simulink model "Hall_sensor_120deg_bare"  (R2024b)
settings: Solver=FixedStepAuto  StartTime=0.0  StopTime=1  FixedStep=1e-6  RelTol=1e-3
values from neighbouring files (symbols this model uses):
  closed_loop = 0    [initialize_model.m]
  D_m = 1e-3    (= 0.001)    [initialize_model.m]
  hall_errors = [0 0 0]    [MTPA_sweep.m]    (also in initialize_model.m = (pi/180)*[-3,5,-4])
  J_t = 12e-4    (= 0.0012)    [initialize_model.m]
  L_ss = 0.45e-3    (= 0.00045)    [Arrow_86EMB3S98F_specs.m]    (also in M_2311P_specs.m = 0.0003657)
  lambda_m = 21.5e-3    (= 0.0215)    [Arrow_86EMB3S98F_specs.m]    (also in M_2311P_specs.m = 0.00985)
  P = 8    [Arrow_86EMB3S98F_specs.m]    (also in M_2311P_specs.m)
  r_s = 0.15    [Arrow_86EMB3S98F_specs.m]    (also in M_2311P_specs.m = 0.345)
  R_vs = 1e6    (= 1000000)    [initialize_model.m]
  T_m = torque_vals(i)    [MTPA_sweep.m]    (also in initialize_model.m = 1.53)
  tau_s = L_ss/r_s    (= 0.003)    [Arrow_86EMB3S98F_specs.m]    (also in M_2311P_specs.m = 0.00106)
  theta_v = pi/6    (= 0.523598775598)    [initialize_model.m]
  V_bus = 36    [initialize_model.m]
undefined symbols (not defined in the file or in its folder): DiscIntNeverNeededParam, dspblkCoreblockFVToolHelper, gcbh, HallError1, HallError2, HallError3, sysd, sysd_mech, WrappedHallError1
libraries: simulink x12, spsMosfetLib x6, spsSeriesRLCBranchLib x4, spsVoltageMeasurementLib x3, spsControlledCurrentSourceLib x3, embmathops x1, spsPWMGeneratorDCDCLib x1, spsDCVoltageSourceLib x1, sps_lib x1
settings Model: Creator=baolo  LastModifiedBy=baolo
settings DebuggingCC: IgnoredZcDiagnostic=none

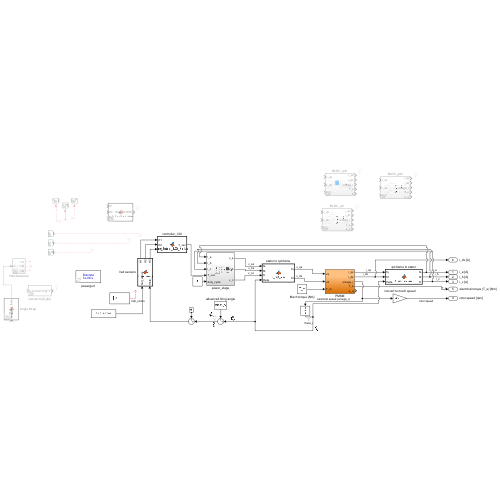
[thumbnail: Simulink's stored preview of the top-level diagram]
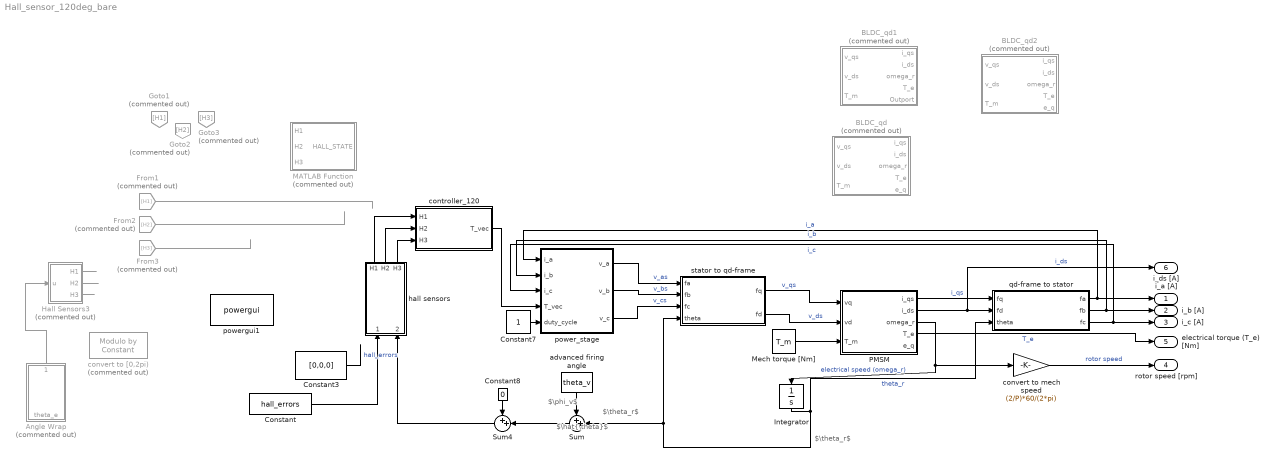
== system Hall_sensor_120deg_bare ==
  note: $\phi_v$
  note: $\theta_r$
  note: $\theta_r$
  note: $\hat{\theta}$
  Angle Wrap : MATLAB Function  Commented=on  TreatAsAtomicUnit=on
  BLDC_qd : Subsystem  Commented=on
  BLDC_qd1 : Subsystem  Commented=on
  BLDC_qd2 : Subsystem  Commented=on
  Constant : Constant  Value=hall_errors
  Constant3 : Constant  Value=[0,0,0]
  Constant7 : Constant
  Constant8 : Constant  Value=0
  From1 : From  Commented=on  GotoTag=H1
  From2 : From  Commented=on  GotoTag=H2
  From3 : From  Commented=on  GotoTag=H3
  Goto1 : Goto  Commented=on  GotoTag=H1
  Goto2 : Goto  Commented=on  GotoTag=H2
  Goto3 : Goto  Commented=on  GotoTag=H3
  Hall Sensors3 : Subsystem  Commented=on
  Integrator : Integrator
  MATLAB Function : MATLAB Function  Commented=on  TreatAsAtomicUnit=on
  Mech torque [Nm] : Constant  Value=T_m
  PMSM : Subsystem
  Sum : Sum  Inputs=++|
  Sum4 : Sum  Inputs=++|
  advanced firing angle : Constant  Value=theta_v
  controller_120 : MATLAB Function  TreatAsAtomicUnit=on
  convert to [0,2pi) : embmathops/Modulo by Constant  Commented=on  Denominator=2*pi  SimulateUsing=Code generation
      settings: LibrarySourceBlock=embeddedMathLib/Modulo by Constant
  convert to mech speed : Gain  Gain=(2/P)*60/(2*pi)
  hall sensors : MATLAB Function  TreatAsAtomicUnit=on
  power_stage : Subsystem
  powergui1 : sps_lib/powergui  Priority=1  SimulationMode=Discrete  SampleTime=1e-6  frequency=60  Iterations=50  frequencyindice=0  Pbase=100e6  ErrMax=1e-4  UnitsV=kV  UnitsW=MW  buscounter=0  FunctionMessages=off  echomessages=off  EnableUseOfTLC=off  CurrentSourceSwitches=off  DisableSnubberDevices=off  DisableRonSwitches=off  DisableVfSwitches=off  DisplayEquations=off  AutomaticDiscreteSolvers=off  SolverType=Tustin/Backward Euler (TBE)  Interpol=off  ExternalGateDelay=off  methode=off  Ts=100  x0status=blocks  SPID=on  SwTol=0  HookPort=off  NonlinearTolerance=1e-4  nMaxIteration=100  ContinueOnMaxIteration=off  RestoreLinks=warning  ResistiveCurrentMeasurement=off  Frange=[0:2:500]  Ylog=off  Xlog=on  ShowGrid=off  save=off  variable=ZData  structure=0  ZoomFFT=off  StartTime=0.0  cycles=1  DisplayStyle=1  fundamental=60  FreqAxis=off  MaxFrequency=1000  frequencyindicesteady=1  RmsSteady=1  display=off
  qd-frame to stator : MATLAB Function  TreatAsAtomicUnit=on
  stator to qd-frame : MATLAB Function  TreatAsAtomicUnit=on
  i_a [A] : Outport
  i_b [A] : Outport  Port=2
  i_c [A] : Outport  Port=3
  rotor speed [rpm] : Outport  Port=4
  electrical torque (T_e) [Nm] : Outport  Port=5
  i_ds [A] : Outport  Port=6
  wires:
  stator to qd-frame/1(fq) -> PMSM/1(vq)  "v_qs"
  stator to qd-frame/2(fd) -> PMSM/2(vd)  "v_ds"
  Mech torque [Nm]/1 -> PMSM/3(T_m)
  PMSM/1(i_qs) -> qd-frame to stator/1(fq)  "i_qs"
  PMSM/2(i_ds) -> i_ds [A]/1, qd-frame to stator/2(fd)  "i_ds"
  PMSM/3(omega_r) -> convert to mech speed/1, Integrator/1  "electrical speed (omega_r)"
  power_stage/1(v_a) -> stator to qd-frame/1(fa)  "v_as"
  power_stage/2(v_b) -> stator to qd-frame/2(fb)  "v_bs"
  power_stage/3(v_c) -> stator to qd-frame/3(fc)  "v_cs"
  Integrator/1 -> stator to qd-frame/4(theta), Sum/2, qd-frame to stator/3(theta)  "theta_r"
  ? -> Goto1/1
  ? -> Goto2/1
  ? -> Goto3/1
  advanced firing angle/1 -> Sum/1
  Sum/1 -> Sum4/2
  qd-frame to stator/1(fa) -> power_stage/1(i_a), i_a [A]/1  "i_a"
  qd-frame to stator/2(fb) -> power_stage/2(i_b), i_b [A]/1  "i_b"
  qd-frame to stator/3(fc) -> power_stage/3(i_c), i_c [A]/1  "i_c"
  convert to mech speed/1 -> rotor speed [rpm]/1  "rotor speed"
  PMSM/4(T_e) -> electrical torque (T_e) [Nm]/1  "T_e"
  Constant3/1 -> ?  "hall_errors"
  controller_120/1(T_vec) -> power_stage/4(T_vec)
  Sum4/1 -> hall sensors/2(theta_r)
  From2/1 -> ?
  From3/1 -> ?
  From1/1 -> ?
  Constant7/1 -> power_stage/5(duty_cycle)
  Constant8/1 -> Sum4/1
  Hall Sensors3/1(H1) -> ?
  Hall Sensors3/2(H2) -> ?
  Hall Sensors3/3(H3) -> ?
  Angle Wrap/1(wrapped_theta) -> Hall Sensors3/1(u)
  hall sensors/1(H1) -> controller_120/1(H1)
  hall sensors/2(H2) -> controller_120/2(H2)
  hall sensors/3(H3) -> controller_120/3(H3)
  Constant/1 -> hall sensors/1(hall_errors)

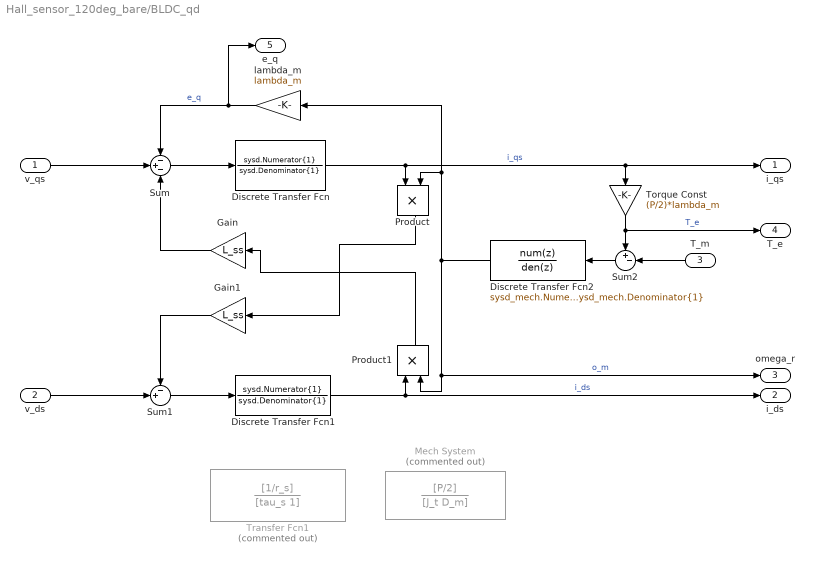
== system Hall_sensor_120deg_bare/BLDC_qd ==
  v_qs : Inport
  v_ds : Inport  Port=2
  T_m : Inport  Port=3
  Discrete Transfer Fcn : DiscreteTransferFcn  LoadFcn=dspblkCoreblockFVToolHelper(gcbh,'load');  Numerator=sysd.Numerator{1}  Denominator=sysd.Denominator{1}  InitialStates=1
      settings: CopyFcn=dspblkCoreblockFVToolHelper(gcbh,'copy');  DeleteFcn=dspblkCoreblockFVToolHelper(gcbh,'close');  ModelCloseFcn=dspblkCoreblockFVToolHelper(gcbh,'close');  PreSaveFcn=dspblkCoreblockFVToolHelper(gcbh,'presave');  PostSaveFcn=dspblkCoreblockFVToolHelper(gcbh,'postsave');  CloseFcn=dspblkCoreblockFVToolHelper(gcbh,'close');
  Discrete Transfer Fcn1 : DiscreteTransferFcn  LoadFcn=dspblkCoreblockFVToolHelper(gcbh,'load');  Numerator=sysd.Numerator{1}  Denominator=sysd.Denominator{1}  InitialStates=1
      settings: CopyFcn=dspblkCoreblockFVToolHelper(gcbh,'copy');  DeleteFcn=dspblkCoreblockFVToolHelper(gcbh,'close');  ModelCloseFcn=dspblkCoreblockFVToolHelper(gcbh,'close');  PreSaveFcn=dspblkCoreblockFVToolHelper(gcbh,'presave');  PostSaveFcn=dspblkCoreblockFVToolHelper(gcbh,'postsave');  CloseFcn=dspblkCoreblockFVToolHelper(gcbh,'close');
  Discrete Transfer Fcn2 : DiscreteTransferFcn  LoadFcn=dspblkCoreblockFVToolHelper(gcbh,'load');  Numerator=sysd_mech.Numerator{1}  Denominator=sysd_mech.Denominator{1}  InitialStates=1
      settings: CopyFcn=dspblkCoreblockFVToolHelper(gcbh,'copy');  DeleteFcn=dspblkCoreblockFVToolHelper(gcbh,'close');  ModelCloseFcn=dspblkCoreblockFVToolHelper(gcbh,'close');  PreSaveFcn=dspblkCoreblockFVToolHelper(gcbh,'presave');  PostSaveFcn=dspblkCoreblockFVToolHelper(gcbh,'postsave');  CloseFcn=dspblkCoreblockFVToolHelper(gcbh,'close');
  Gain : Gain  Gain=L_ss
  Gain1 : Gain  Gain=L_ss
  Mech System : TransferFcn  Commented=on  Numerator=[P/2]  Denominator=[J_t D_m]
  Product : Product
  Product1 : Product
  Sum : Sum  Inputs=-+-
  Sum1 : Sum  Inputs=-+|
  Sum2 : Sum  Inputs=+-|
  Torque Const : Gain  Gain=(P/2)*lambda_m
  Transfer Fcn1 : TransferFcn  Commented=on  Numerator=[1/r_s]  Denominator=[tau_s 1]
  lambda_m : Gain  Gain=lambda_m
  i_qs : Outport
  i_ds : Outport  Port=2
  omega_r : Outport  Port=3
  T_e : Outport  Port=4
  e_q : Outport  Port=5
  wires:
  T_m/1 -> Sum2/2
  Sum1/1 -> Discrete Transfer Fcn1/1
  Gain1/1 -> Sum1/1
  Product1/1 -> Gain/1
  Discrete Transfer Fcn1/1 -> i_ds/1, Product1/1  "i_ds"
  Discrete Transfer Fcn2/1 -> lambda_m/1, Product/2, omega_r/1, Product1/2  "o_m"
  Torque Const/1 -> T_e/1, Sum2/1  "T_e"
  v_ds/1 -> Sum1/2
  Discrete Transfer Fcn/1 -> i_qs/1, Torque Const/1, Product/1  "i_qs"
  Product/1 -> Gain1/1
  Gain/1 -> Sum/3
  v_qs/1 -> Sum/2
  Sum/1 -> Discrete Transfer Fcn/1
  Sum2/1 -> Discrete Transfer Fcn2/1
  lambda_m/1 -> e_q/1, Sum/1  "e_q"

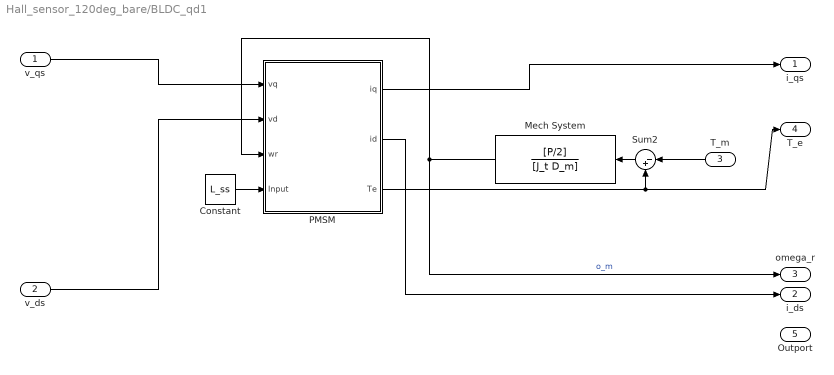
== system Hall_sensor_120deg_bare/BLDC_qd1 ==
  v_qs : Inport
  v_ds : Inport  Port=2
  T_m : Inport  Port=3
  Constant : Constant  Value=L_ss
  Mech System : TransferFcn  Numerator=[P/2]  Denominator=[J_t D_m]
  PMSM : Subsystem
  Sum2 : Sum  Inputs=|-+
  i_qs : Outport
  i_ds : Outport  Port=2
  omega_r : Outport  Port=3
  T_e : Outport  Port=4
  Outport : Outport  Port=5
  wires:
  T_m/1 -> Sum2/1
  Sum2/1 -> Mech System/1
  v_qs/1 -> PMSM/1(vq)
  v_ds/1 -> PMSM/2(vd)
  Constant/1 -> PMSM/4(Input)
  Mech System/1 -> omega_r/1, PMSM/3(wr)  "o_m"
  PMSM/1(iq) -> i_qs/1
  PMSM/2(id) -> i_ds/1
  PMSM/3(Te) -> Sum2/2, T_e/1

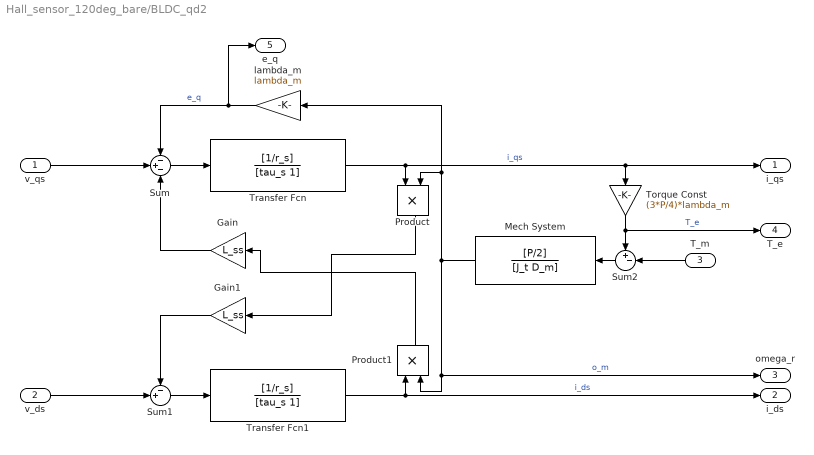
== system Hall_sensor_120deg_bare/BLDC_qd2 ==
  v_qs : Inport
  v_ds : Inport  Port=2
  T_m : Inport  Port=3
  Gain : Gain  Gain=L_ss
  Gain1 : Gain  Gain=L_ss
  Mech System : TransferFcn  Numerator=[P/2]  Denominator=[J_t D_m]
  Product : Product
  Product1 : Product
  Sum : Sum  Inputs=-+-
  Sum1 : Sum  Inputs=-+|
  Sum2 : Sum  Inputs=+-|
  Torque Const : Gain  Gain=(3*P/4)*lambda_m
  Transfer Fcn : TransferFcn  Numerator=[1/r_s]  Denominator=[tau_s 1]
  Transfer Fcn1 : TransferFcn  Numerator=[1/r_s]  Denominator=[tau_s 1]
  lambda_m : Gain  Gain=lambda_m
  i_qs : Outport
  i_ds : Outport  Port=2
  omega_r : Outport  Port=3
  T_e : Outport  Port=4
  e_q : Outport  Port=5
  wires:
  T_m/1 -> Sum2/2
  Sum1/1 -> Transfer Fcn1/1
  Gain1/1 -> Sum1/1
  Product1/1 -> Gain/1
  Transfer Fcn1/1 -> i_ds/1, Product1/1  "i_ds"
  Mech System/1 -> lambda_m/1, Product/2, omega_r/1, Product1/2  "o_m"
  Torque Const/1 -> T_e/1, Sum2/1  "T_e"
  v_ds/1 -> Sum1/2
  Transfer Fcn/1 -> i_qs/1, Torque Const/1, Product/1  "i_qs"
  Product/1 -> Gain1/1
  Gain/1 -> Sum/3
  v_qs/1 -> Sum/2
  Sum/1 -> Transfer Fcn/1
  Sum2/1 -> Mech System/1
  lambda_m/1 -> e_q/1, Sum/1  "e_q"

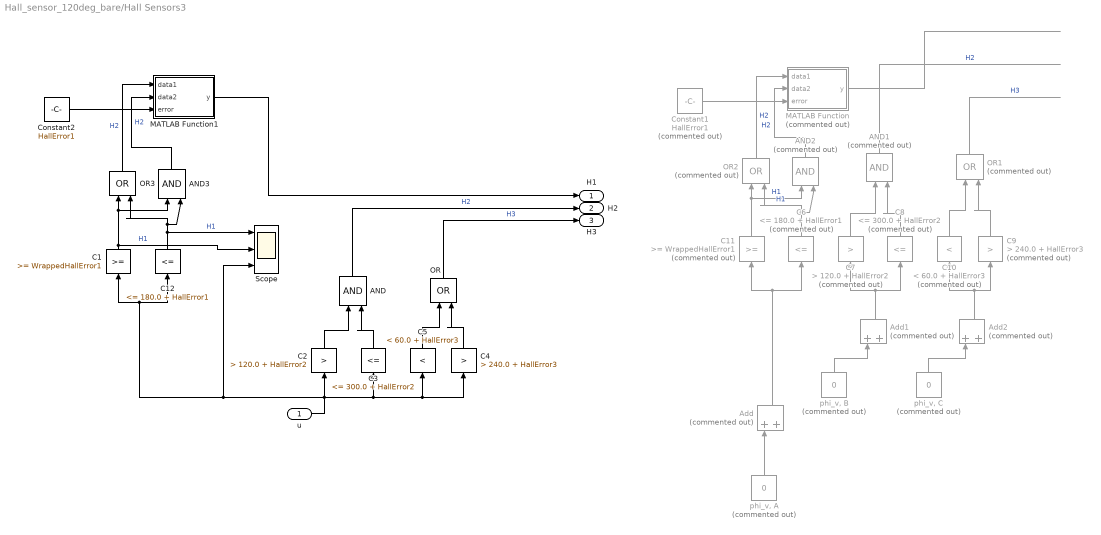
== system Hall_sensor_120deg_bare/Hall Sensors3 ==
  u : Inport
  AND : Logic  IconShape=distinctive  AllPortsSameDT=off  OutDataTypeStr=boolean
  AND1 : Logic  Commented=on  IconShape=distinctive  AllPortsSameDT=off  OutDataTypeStr=boolean
  AND2 : Logic  Commented=on  IconShape=distinctive  AllPortsSameDT=off  OutDataTypeStr=boolean
  AND3 : Logic  IconShape=distinctive  AllPortsSameDT=off  OutDataTypeStr=boolean
  Add : Sum  Commented=on
  Add1 : Sum  Commented=on
  Add2 : Sum  Commented=on
  C1 : simulink/Logic and Bit Operations/Compare To Constant  relop=>=  const=WrappedHallError1  OutDataTypeStr=boolean
  C10 : simulink/Logic and Bit Operations/Compare To Constant  Commented=on  relop=<  const=60.0 + HallError3  OutDataTypeStr=boolean
  C11 : simulink/Logic and Bit Operations/Compare To Constant  Commented=on  relop=>=  const=WrappedHallError1  OutDataTypeStr=boolean
  C12 : simulink/Logic and Bit Operations/Compare To Constant  relop=<=  const=180.0 + HallError1  OutDataTypeStr=boolean
  C2 : simulink/Logic and Bit Operations/Compare To Constant  relop=>  const=120.0 + HallError2  OutDataTypeStr=boolean
  C3 : simulink/Logic and Bit Operations/Compare To Constant  relop=<=  const=300.0 + HallError2  OutDataTypeStr=boolean
  C4 : simulink/Logic and Bit Operations/Compare To Constant  relop=>  const=240.0 + HallError3  OutDataTypeStr=boolean
  C5 : simulink/Logic and Bit Operations/Compare To Constant  relop=<  const=60.0 + HallError3  OutDataTypeStr=boolean
  C6 : simulink/Logic and Bit Operations/Compare To Constant  Commented=on  relop=<=  const=180.0 + HallError1  OutDataTypeStr=boolean
  C7 : simulink/Logic and Bit Operations/Compare To Constant  Commented=on  relop=>  const=120.0 + HallError2  OutDataTypeStr=boolean
  C8 : simulink/Logic and Bit Operations/Compare To Constant  Commented=on  relop=<=  const=300.0 + HallError2  OutDataTypeStr=boolean
  C9 : simulink/Logic and Bit Operations/Compare To Constant  Commented=on  relop=>  const=240.0 + HallError3  OutDataTypeStr=boolean
  Constant1 : Constant  Commented=on  Value=HallError1
  Constant2 : Constant  Value=HallError1
  MATLAB Function : MATLAB Function  Commented=on  TreatAsAtomicUnit=on
  MATLAB Function1 : MATLAB Function  TreatAsAtomicUnit=on
  OR : Logic  Operator=OR  IconShape=distinctive  AllPortsSameDT=off  OutDataTypeStr=boolean
  OR1 : Logic  Commented=on  Operator=OR  IconShape=distinctive  AllPortsSameDT=off  OutDataTypeStr=boolean
  OR2 : Logic  Commented=on  Operator=OR  IconShape=distinctive  AllPortsSameDT=off  OutDataTypeStr=boolean
  OR3 : Logic  Operator=OR  IconShape=distinctive  AllPortsSameDT=off  OutDataTypeStr=boolean
  Scope : Scope  NumInputPorts=3
  "phi_v, A" : Constant  Commented=on  Value=0
  "phi_v, B" : Constant  Commented=on  Value=0
  "phi_v, C" : Constant  Commented=on  Value=0
  H1 : Outport
  H2 : Outport  Port=2
  H3 : Outport  Port=3
  wires:
  C5/1 -> OR/1
  AND/1 -> H2/1  "H2"
  C4/1 -> OR/2
  C3/1 -> AND/2
  C2/1 -> AND/1
  OR/1 -> H3/1  "H3"
  Add1/1 -> C8/1, C7/1
  "phi_v, C"/1 -> Add2/1
  "phi_v, B"/1 -> Add1/1
  C10/1 -> OR1/1
  ? -> Add2/2, Add1/2, Add/2
  OR2/1 -> MATLAB Function/1(data1)  "H2"
  "phi_v, A"/1 -> Add/1
  C9/1 -> OR1/2
  Add/1 -> C6/1, C11/1
  C7/1 -> AND1/1
  Add2/1 -> C10/1, C9/1
  Constant1/1 -> MATLAB Function/3(error)
  OR1/1 -> ?  "H3"
  AND1/1 -> ?  "H2"
  C6/1 -> AND2/2, OR2/2  "H1"
  AND2/1 -> MATLAB Function/2(data2)  "H2"
  MATLAB Function/1(y) -> ?
  C11/1 -> AND2/1, OR2/1  "H1"
  C8/1 -> AND1/2
  u/1 -> Scope/3, C12/1, C1/1, C2/1, C5/1, C4/1, C3/1
  OR3/1 -> MATLAB Function1/1(data1)  "H2"
  Constant2/1 -> MATLAB Function1/3(error)
  C1/1 -> AND3/1, OR3/1, Scope/2  "H1"
  C12/1 -> AND3/2, OR3/2, Scope/1  "H1"
  AND3/1 -> MATLAB Function1/2(data2)  "H2"
  MATLAB Function1/1(y) -> H1/1

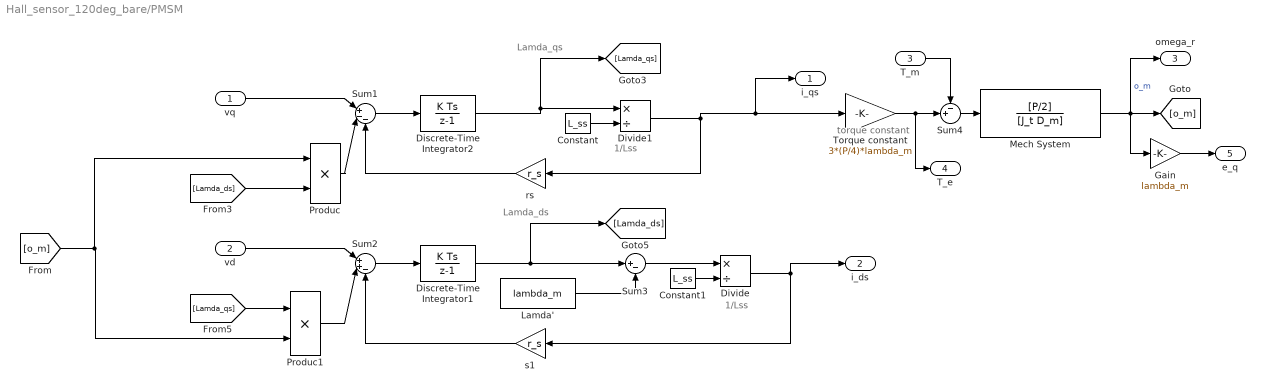
== system Hall_sensor_120deg_bare/PMSM ==
  note: torque constant
  note: Lamda_ds
  note: Lamda_qs
  note: 1/Lss
  note: 1/Lss
  vq : Inport
  vd : Inport  Port=2
  T_m : Inport  Port=3
  Constant : Constant  Value=L_ss
  Constant1 : Constant  Value=L_ss
  Discrete-Time Integrator1 : DiscreteIntegrator  SampleTime=-1  ICPrevOutput=DiscIntNeverNeededParam  ICPrevScaledInput=DiscIntNeverNeededParam
  Discrete-Time Integrator2 : DiscreteIntegrator  SampleTime=-1  ICPrevOutput=DiscIntNeverNeededParam  ICPrevScaledInput=DiscIntNeverNeededParam
  Divide : Product  Inputs=*/
  Divide1 : Product  Inputs=*/
  Gain : Gain  Gain=lambda_m
  Lamda' : Constant  Value=lambda_m
  Mech System : TransferFcn  Numerator=[P/2]  Denominator=[J_t D_m]
  Produc : Product  RndMeth=Zero
  Produc1 : Product  RndMeth=Zero
  Sum1 : Sum  Inputs=|+--
  Sum2 : Sum  Inputs=|++-
  Sum3 : Sum  Inputs=|+-
  Sum4 : Sum  Inputs=-+|
  Torque constant : Gain  Gain=3*(P/4)*lambda_m
  rs : Gain  Gain=r_s
  s1 : Gain  Gain=r_s
  i_qs : Outport
  i_ds : Outport  Port=2
  omega_r : Outport  Port=3
  T_e : Outport  Port=4
  e_q : Outport  Port=5
  wires:
  vd/1 -> Sum2/1
  vq/1 -> Sum1/1
  [Lamda_qs] -> Produc1/1
  [Lamda_ds] -> Produc/2
  [o_m] -> Produc1/2, Produc/1
  Lamda'/1 -> Sum3/2
  Sum3/1 -> Divide/1
  s1/1 -> Sum2/3
  Discrete-Time Integrator1/1 -> [Lamda_ds], Sum3/1
  Sum2/1 -> Discrete-Time Integrator1/1
  Produc1/1 -> Sum2/2
  Divide1/1 -> i_qs/1, Torque constant/1, rs/1
  rs/1 -> Sum1/3
  Discrete-Time Integrator2/1 -> [Lamda_qs], Divide1/1
  Sum1/1 -> Discrete-Time Integrator2/1
  Produc/1 -> Sum1/2
  Torque constant/1 -> Sum4/2, T_e/1
  Divide/1 -> i_ds/1, s1/1
  T_m/1 -> Sum4/1
  Sum4/1 -> Mech System/1
  Constant/1 -> Divide1/2
  Constant1/1 -> Divide/2
  Mech System/1 -> Gain/1, omega_r/1, [o_m]  "o_m"
  Gain/1 -> e_q/1

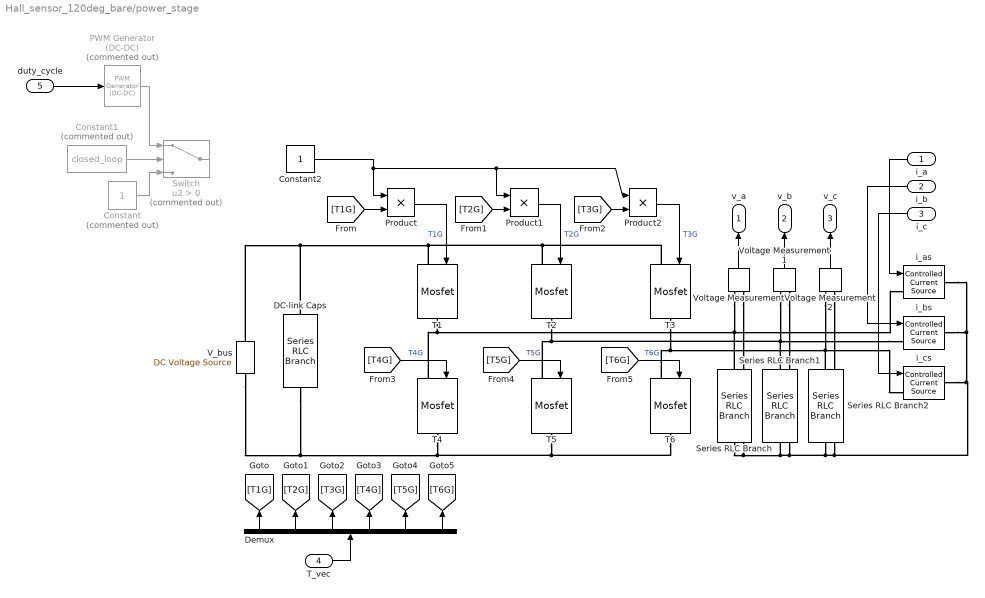
== system Hall_sensor_120deg_bare/power_stage ==
  i_a : Inport
  i_b : Inport  Port=2
  i_c : Inport  Port=3
  T_vec : Inport  Port=4
  duty_cycle : Inport  Port=5
  Constant : Constant  Commented=on
  Constant1 : Constant  Commented=on  Value=closed_loop
  Constant2 : Constant
  DC-link Caps : spsSeriesRLCBranchLib/Series RLC Branch  LConnTagsString=__new0  RConnTagsString=__new0  BranchType=RC  Resistance=1e-6  Inductance=0  SetiL0=off  InitialCurrent=0  Capacitance=100e-6  Setx0=off  InitialVoltage=0  Measurements=None
  Demux : Demux  Outputs=6
  PWM Generator (DC-DC) : spsPWMGeneratorDCDCLib/PWM Generator (DC-DC)  Commented=on  Fsw=f_SW_Hz  Ts=0
  Product : Product
  Product1 : Product
  Product2 : Product
  Series RLC Branch : spsSeriesRLCBranchLib/Series RLC Branch  LConnTagsString=__new0  RConnTagsString=__new0  BranchType=R  Resistance=R_vs  Inductance=0  SetiL0=off  InitialCurrent=0  Capacitance=inf  Setx0=off  InitialVoltage=0  Measurements=None
  Series RLC Branch1 : spsSeriesRLCBranchLib/Series RLC Branch  LConnTagsString=__new0  RConnTagsString=__new0  BranchType=R  Resistance=R_vs  Inductance=0  SetiL0=off  InitialCurrent=0  Capacitance=inf  Setx0=off  InitialVoltage=0  Measurements=None
  Series RLC Branch2 : spsSeriesRLCBranchLib/Series RLC Branch  LConnTagsString=__new0  RConnTagsString=__new0  BranchType=R  Resistance=R_vs  Inductance=0  SetiL0=off  InitialCurrent=0  Capacitance=inf  Setx0=off  InitialVoltage=0  Measurements=None
  Switch : Switch  Commented=on  Criteria=u2 > Threshold  SaturateOnIntegerOverflow=off  InputSameDT=off
  T{1..6} (6 alike) : spsMosfetLib/Mosfet  Ron=R_dsON_Ohm  Lon=0  Rd=0.01  Vfd=0.7  IC=0  Rs=1e5  Cs=inf  Measurements=off
  V_bus : spsDCVoltageSourceLib/DC Voltage Source  Amplitude=V_bus  Measurements=None
  Voltage Measurement : spsVoltageMeasurementLib/Voltage Measurement  PhasorSimulation=off  OutputType=Complex  PSBequivalent=0
  Voltage Measurement1 : spsVoltageMeasurementLib/Voltage Measurement  PhasorSimulation=off  OutputType=Complex  PSBequivalent=0
  Voltage Measurement2 : spsVoltageMeasurementLib/Voltage Measurement  PhasorSimulation=off  OutputType=Complex  PSBequivalent=0
  i_as : spsControlledCurrentSourceLib/Controlled Current Source  Initialize=on  Source_Type=AC  Amplitude=0  Phase=0  Frequency=0  Measurements=None
  i_bs : spsControlledCurrentSourceLib/Controlled Current Source  Initialize=on  Source_Type=AC  Amplitude=0  Phase=0  Frequency=0  Measurements=None
  i_cs : spsControlledCurrentSourceLib/Controlled Current Source  Initialize=on  Source_Type=AC  Amplitude=0  Phase=0  Frequency=0  Measurements=None
  v_a : Outport
  v_b : Outport  Port=2
  v_c : Outport  Port=3
  wires:
  T_vec/1 -> Demux/1
  Product1/1 -> T2/1  "T2G"
  Constant2/1 -> Product/1, Product2/1, Product1/1
  Demux/6 -> [T6G]
  [T4G] -> T4/1  "T4G"
  [T5G] -> T5/1  "T5G"
  Demux/4 -> [T4G]
  Voltage Measurement/1 -> v_a/1
  [T2G] -> Product1/2
  Voltage Measurement1/1 -> v_b/1
  Voltage Measurement2/1 -> v_c/1
  i_a/1 -> i_as/1
  Demux/1 -> [T1G]
  Demux/5 -> [T5G]
  [T6G] -> T6/1  "T6G"
  i_c/1 -> i_cs/1
  Product/1 -> T1/1  "T1G"
  [T3G] -> Product2/2
  i_b/1 -> i_bs/1
  Product2/1 -> T3/1  "T3G"
  Demux/2 -> [T2G]
  Demux/3 -> [T3G]
  [T1G] -> Product/2
  duty_cycle/1 -> PWM Generator (DC-DC)/1
  Constant/1 -> Switch/3
  Constant1/1 -> Switch/2
  PWM Generator (DC-DC)/1 -> Switch/1
  connections:
  i_bs/LConn1 -- Voltage Measurement1/LConn1 -- Series RLC Branch1/LConn1 -- T2/RConn1 -- T5/LConn1
  DC-link Caps/RConn1 -- V_bus/LConn1 -- T4/RConn1 -- T6/RConn1 -- T5/RConn1
  DC-link Caps/LConn1 -- V_bus/RConn1 -- T1/LConn1 -- T3/LConn1 -- T2/LConn1
  T4/LConn1 -- T1/RConn1 -- Voltage Measurement/LConn1 -- Series RLC Branch/LConn1 -- i_as/LConn1
  T3/RConn1 -- T6/LConn1 -- Voltage Measurement2/LConn1 -- Series RLC Branch2/LConn1 -- i_cs/LConn1
  Series RLC Branch/RConn1 -- Voltage Measurement/LConn2 -- i_bs/RConn1 -- i_as/RConn1 -- i_cs/RConn1 -- Voltage Measurement2/LConn2 -- Series RLC Branch2/RConn1 -- Voltage Measurement1/LConn2 -- Series RLC Branch1/RConn1

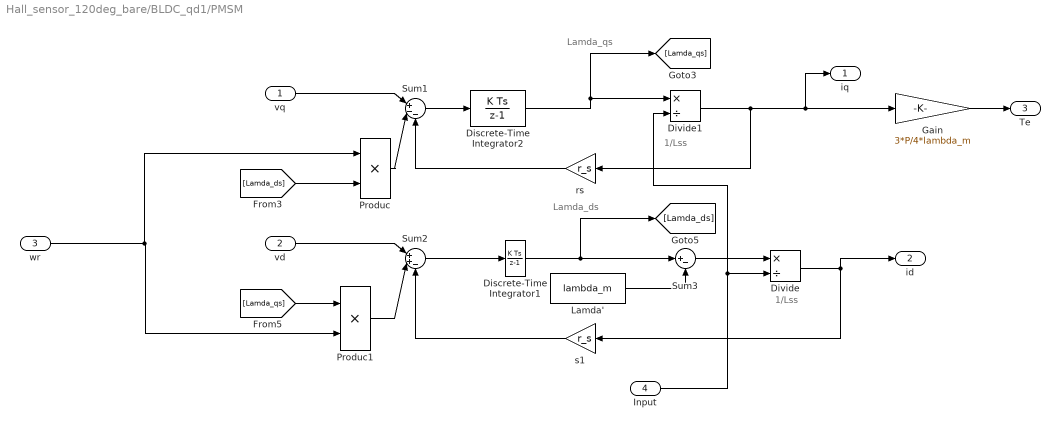
== system Hall_sensor_120deg_bare/BLDC_qd1/PMSM ==
  note: Lamda_ds
  note: Lamda_qs
  note: 1/Lss
  note: 1/Lss
  vq : Inport
  vd : Inport  Port=2
  wr : Inport  Port=3
  Input : Inport  Port=4
  Discrete-Time Integrator1 : DiscreteIntegrator  SampleTime=-1  ICPrevOutput=DiscIntNeverNeededParam  ICPrevScaledInput=DiscIntNeverNeededParam
  Discrete-Time Integrator2 : DiscreteIntegrator  SampleTime=-1  ICPrevOutput=DiscIntNeverNeededParam  ICPrevScaledInput=DiscIntNeverNeededParam
  Divide : Product  Inputs=*/
  Divide1 : Product  Inputs=*/
  Gain : Gain  Gain=3*P/4*lambda_m
  Lamda' : Constant  Value=lambda_m
  Produc : Product  RndMeth=Zero
  Produc1 : Product  RndMeth=Zero
  Sum1 : Sum  Inputs=|+--
  Sum2 : Sum  Inputs=|++-
  Sum3 : Sum  Inputs=|+-
  rs : Gain  Gain=r_s
  s1 : Gain  Gain=r_s
  iq : Outport
  id : Outport  Port=2
  Te : Outport  Port=3
  wires:
  vd/1 -> Sum2/1
  vq/1 -> Sum1/1
  [Lamda_qs] -> Produc1/1
  [Lamda_ds] -> Produc/2
  wr/1 -> Produc1/2, Produc/1
  Lamda'/1 -> Sum3/2
  Sum3/1 -> Divide/1
  s1/1 -> Sum2/3
  Discrete-Time Integrator1/1 -> [Lamda_ds], Sum3/1
  Sum2/1 -> Discrete-Time Integrator1/1
  Produc1/1 -> Sum2/2
  Divide1/1 -> rs/1, Gain/1, iq/1
  rs/1 -> Sum1/3
  Discrete-Time Integrator2/1 -> Divide1/1, [Lamda_qs]
  Sum1/1 -> Discrete-Time Integrator2/1
  Produc/1 -> Sum1/2
  Gain/1 -> Te/1
  Divide/1 -> id/1, s1/1
  Input/1 -> Divide/2, Divide1/2

== matlab function Hall_sensor_120deg_bare/qd-frame to stator ==
  data: fa output; fb output; fc output; fq input; fd input; theta input
function [fa,fb,fc] = K_mat_inv_sim(fq,fd,theta)
[fa,fb,fc] = K_mat_inv(fq,fd,theta);

== matlab function Hall_sensor_120deg_bare/stator to qd-frame ==
  data: fa input; fq output; fb input; fc input; theta input; fd output
function [fq,fd] = K_mat_sim(fa,fb,fc,theta)
[fq,fd] = K_mat(fa,fb,fc,theta);

== matlab function Hall_sensor_120deg_bare/hall sensors ==
  data: hall_errors input; theta_r input; H1 output; H2 output; H3 output
function [H1,H2,H3] = hall_sensor_sim(hall_errors, theta_r)
[H1,H2,H3] = hall_sensor(theta_r, hall_errors);
end

== matlab function Hall_sensor_120deg_bare/controller_120 ==
  data: H1 input; T_vec output; H2 input; H3 input
function T_vec = controller_6step_120_hallvec_sim(H1,H2,H3)
T_vec = controller_6step_120_hallvec(H1,H2,H3);
end

== matlab function Hall_sensor_120deg_bare/MATLAB Function ==
  data: H1 input; HALL_STATE output; H2 input; H3 input
function HALL_STATE = hall_to_statenum(H1,H2,H3)
HALL_STATE = 4*H1 + 2*H2 + H3;

== matlab function Hall_sensor_120deg_bare/Angle Wrap ==
  data: theta_e input; wrapped_theta output
function wrapped_theta = fcn(theta_e)

wrapped_theta = wrapTo2Pi(theta_e) * 180 / pi;

== matlab function Hall_sensor_120deg_bare/Hall Sensors3/MATLAB Function ==
  data: data1 input; y output; data2 input; error input
function y = fcn(data1, data2, error)

if error > 0
    y = data2;

else 
    y = data1;

end

== matlab function Hall_sensor_120deg_bare/Hall Sensors3/MATLAB Function1 ==
  data: data1 input; y output; data2 input; error input
function y = fcn(data1, data2, error)

if error > 0
    y = data2;

else 
    y = data1;

end
